simulink model "AM"  (R2014b)
settings: Solver=ode45  StartTime=0.0  StopTime=10.0  RelTol=1e-3
libraries: dsparch4 x1, commnoisgen2 x1
settings Model: Creator=TY  LastModifiedBy=TY

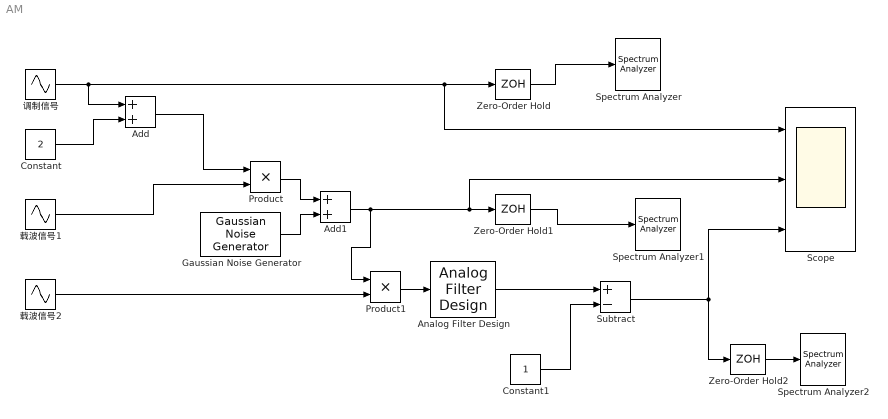
== system AM ==
  Add : Sum
  Add1 : Sum
  Analog Filter Design : dsparch4/Analog Filter Design  method=Butterworth  filttype=Lowpass  N=8  Wlo=25*6.28  Whi=80  Rp=2  Rs=40
  Constant : Constant  Value=2
  Constant1 : Constant
  Gaussian Noise Generator : commnoisgen2/Gaussian Noise Generator  m=0  d=0  s=41  Ts=1/10000  frameBased=off  sampPerFrame=1  orient=off  outDataType=double
  Product : Product
  Product1 : Product
  Scope : Scope  NumInputPorts=3
      settings: TimeRange=9.992710929977697  YMin=-1~-3~-1  YMax=1~3~1
  Spectrum Analyzer : SpectrumAnalyzer
  Spectrum Analyzer1 : SpectrumAnalyzer
  Spectrum Analyzer2 : SpectrumAnalyzer
  Subtract : Sum  Inputs=+-
  Zero-Order Hold : ZeroOrderHold  SampleTime=1/1000
  Zero-Order Hold1 : ZeroOrderHold  SampleTime=1/1000
  Zero-Order Hold2 : ZeroOrderHold  SampleTime=1/1000
  调制信号 : Sin  Frequency=20*6.28  SampleTime=0
  载波信号1 : Sin  Frequency=200*6.28  SampleTime=0
  载波信号2 : Sin  Frequency=200*6.28  SampleTime=0
  wires:
  调制信号/1 -> Add/1, Scope/1, Zero-Order Hold/1
  Add/1 -> Product/1
  Product1/1 -> Analog Filter Design/1
  Analog Filter Design/1 -> Subtract/1
  Subtract/1 -> Scope/3, Zero-Order Hold2/1
  Constant/1 -> Add/2
  Zero-Order Hold/1 -> Spectrum Analyzer/1
  Constant1/1 -> Subtract/2
  Zero-Order Hold1/1 -> Spectrum Analyzer1/1
  载波信号2/1 -> Product1/2
  载波信号1/1 -> Product/2
  Zero-Order Hold2/1 -> Spectrum Analyzer2/1
  Product/1 -> Add1/1
  Gaussian Noise Generator/1 -> Add1/2
  Add1/1 -> Product1/1, Scope/2, Zero-Order Hold1/1
